simulink model "sim_modelo_dinamico_lineal"  (R2019b)
settings: Solver=VariableStepAuto  StartTime=0.0  StopTime=1.0  RelTol=1e-3
undefined symbols (not defined in the file or in its folder): denq1, numq1
settings Model: Creator=AlejnadroZapett  LastModifiedBy=AlejnadroZapett

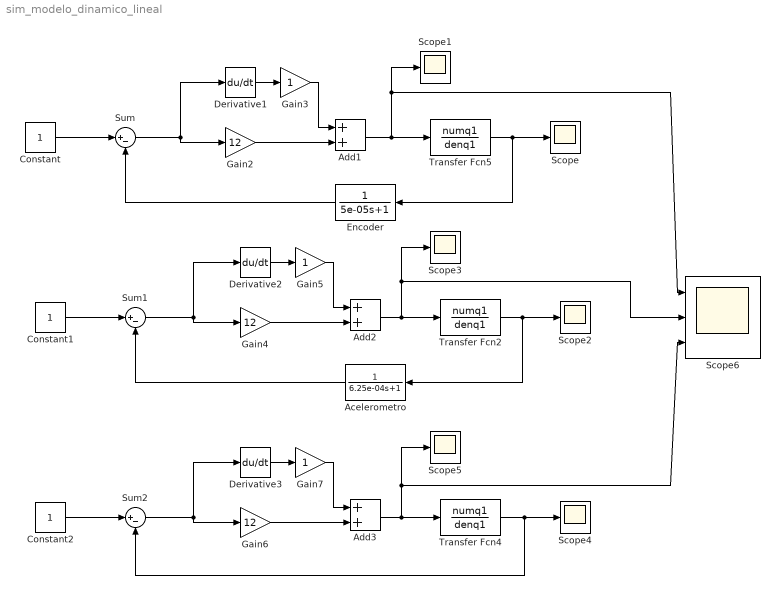
== system sim_modelo_dinamico_lineal ==
  Acelerometro : TransferFcn  Denominator=[6.25e-04 1]
  Add1 : Sum
  Add2 : Sum
  Add3 : Sum
  Constant : Constant
  Constant1 : Constant
  Constant2 : Constant
  Derivative1 : Derivative
  Derivative2 : Derivative
  Derivative3 : Derivative
  Encoder : TransferFcn  Denominator=[5e-05 1]
  Gain2 : Gain  Gain=12
  Gain3 : Gain
  Gain4 : Gain  Gain=12
  Gain5 : Gain
  Gain6 : Gain  Gain=12
  Gain7 : Gain
  Scope{,1..5} (6 alike) : Scope
  Scope6 : Scope  NumInputPorts=3
  Sum : Sum  Inputs=|+-
  Sum1 : Sum  Inputs=|+-
  Sum2 : Sum  Inputs=|+-
  Transfer Fcn2 : TransferFcn  Numerator=numq1  Denominator=denq1
  Transfer Fcn4 : TransferFcn  Numerator=numq1  Denominator=denq1
  Transfer Fcn5 : TransferFcn  Numerator=numq1  Denominator=denq1
  wires:
  Sum/1 -> Derivative1/1, Gain2/1
  Constant/1 -> Sum/1
  Encoder/1 -> Sum/2
  Transfer Fcn5/1 -> Scope/1, Encoder/1
  Add1/1 -> Transfer Fcn5/1, Scope6/1, Scope1/1
  Constant1/1 -> Sum1/1
  Add2/1 -> Transfer Fcn2/1, Scope3/1, Scope6/2
  Transfer Fcn2/1 -> Scope2/1, Acelerometro/1
  Acelerometro/1 -> Sum1/2
  Sum2/1 -> Derivative3/1, Gain6/1
  Constant2/1 -> Sum2/1
  Add3/1 -> Scope6/3, Scope5/1, Transfer Fcn4/1
  Transfer Fcn4/1 -> Sum2/2, Scope4/1
  ? -> ?
  Gain3/1 -> Add1/1
  Gain2/1 -> Add1/2
  Derivative1/1 -> Gain3/1
  Gain5/1 -> Add2/1
  Gain4/1 -> Add2/2
  Derivative2/1 -> Gain5/1
  Sum1/1 -> Derivative2/1, Gain4/1
  Gain7/1 -> Add3/1
  Gain6/1 -> Add3/2
  Derivative3/1 -> Gain7/1
